simulink model "DLCI"  (R2023b)
settings: Solver=FixedStepDiscrete  StartTime=0.0  StopTime=10.0  FixedStep=0.01  RelTol=1e-3
settings Model: Creator=LENOVO-MCC  LastModifiedBy=LENOVO-MCC
settings OptimizationCC: DefaultParameterBehavior=Inlined  EnhancedBackFolding=on  PassReuseOutputArgsAs=Individual arguments  ZeroExternalMemoryAtStartup=off  ZeroInternalMemoryAtStartup=off  OptimizeBlockOrder=speed  DifferentSizesBufferReuse=on  OptimizationCustomize=off  EfficientTunableParamExpr=on
settings DebuggingCC: ParameterTunabilityLossMsg=error
settings SFSimCC: MATLABDynamicMemAlloc=off
settings RTWCC: Description=Embedded Coder  SystemTargetFile=ert.tlc  GenCodeOnly=on  TemplateMakefile=ert_default_tmf  GenerateReport=on  LaunchReport=on  GenerateCodeMetricsReport=on
settings CodeAppCC: ForceParamTrailComments=on  IgnoreCustomStorageClasses=off  OperatorAnnotations=on  SimulinkDataObjDesc=on  SFDataObjDesc=on  InsertBlockDesc=on
settings ERTTargetCC: TargetLangStandard=C99 (ISO)  GenerateSampleERTMain=on  InlinedParameterPlacement=NonHierarchical  ERTCustomFileTemplate=example_file_process.tlc

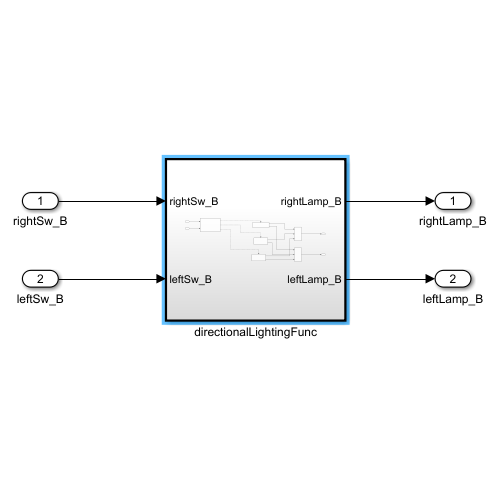
[thumbnail: Simulink's stored preview of the top-level diagram]
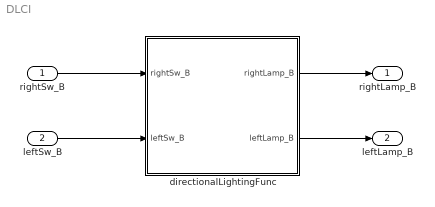
== system DLCI ==
  rightSw_B : Inport  OutDataTypeStr=boolean
  leftSw_B : Inport  Port=2  OutDataTypeStr=boolean
  directionalLightingFunc : Subsystem  TreatAsAtomicUnit=on
      settings: RTWFcnNameOpts=Use subsystem name  RTWFileNameOpts=Use subsystem name
  rightLamp_B : Outport  OutDataTypeStr=boolean
  leftLamp_B : Outport  Port=2  OutDataTypeStr=boolean
  wires:
  leftSw_B/1 -> directionalLightingFunc/2(leftSw_B)
  rightSw_B/1 -> directionalLightingFunc/1(rightSw_B)
  directionalLightingFunc/1(rightLamp_B) -> rightLamp_B/1
  directionalLightingFunc/2(leftLamp_B) -> leftLamp_B/1

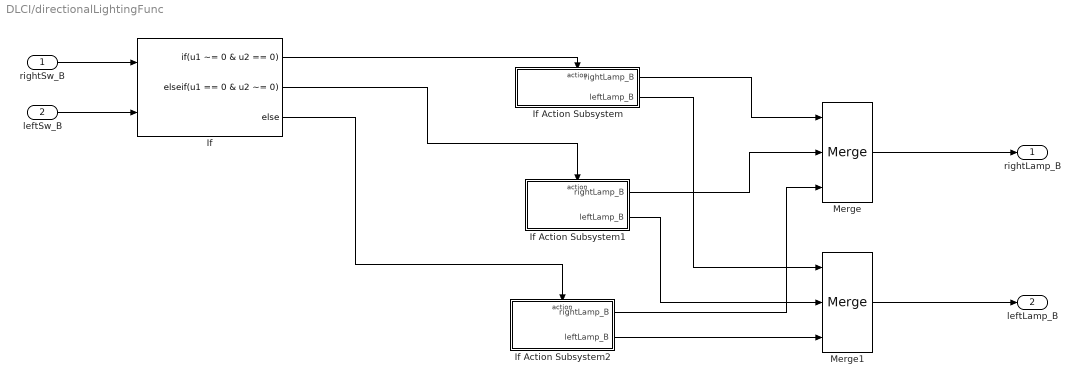
== system DLCI/directionalLightingFunc ==
  rightSw_B : Inport  OutDataTypeStr=boolean
  leftSw_B : Inport  Port=2  OutDataTypeStr=boolean
  If : If  NumInputs=2  IfExpression=u1 ~= 0 & u2 == 0  ElseIfExpressions=u1 == 0 & u2 ~= 0
  If Action Subsystem : Subsystem  TreatAsAtomicUnit=on
  If Action Subsystem1 : Subsystem  TreatAsAtomicUnit=on
  If Action Subsystem2 : Subsystem  TreatAsAtomicUnit=on
  Merge : Merge  Inputs=3
  Merge1 : Merge  Inputs=3
  rightLamp_B : Outport  OutDataTypeStr=boolean
  leftLamp_B : Outport  Port=2  OutDataTypeStr=boolean
  wires:
  rightSw_B/1 -> If/1
  leftSw_B/1 -> If/2
  If/1 -> If Action Subsystem/Action
  If/2 -> If Action Subsystem1/Action
  If/3 -> If Action Subsystem2/Action
  If Action Subsystem/1(rightLamp_B) -> Merge/1
  If Action Subsystem1/1(rightLamp_B) -> Merge/2
  If Action Subsystem2/1(rightLamp_B) -> Merge/3
  Merge/1 -> rightLamp_B/1
  Merge1/1 -> leftLamp_B/1
  If Action Subsystem/2(leftLamp_B) -> Merge1/1
  If Action Subsystem1/2(leftLamp_B) -> Merge1/2
  If Action Subsystem2/2(leftLamp_B) -> Merge1/3

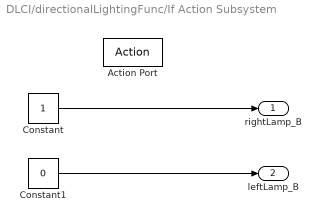
== system DLCI/directionalLightingFunc/If Action Subsystem ==
  Action Port : ActionPort  ActionPortLabel=if(u1 ~= 0 & u2 == 0)
  Constant : Constant  OutDataTypeStr=boolean
  Constant1 : Constant  Value=0  OutDataTypeStr=boolean
  rightLamp_B : Outport
  leftLamp_B : Outport  Port=2
  wires:
  Constant/1 -> rightLamp_B/1
  Constant1/1 -> leftLamp_B/1

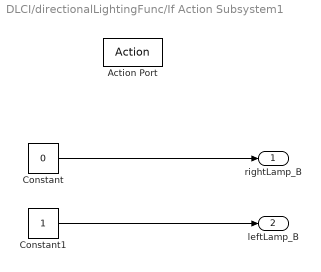
== system DLCI/directionalLightingFunc/If Action Subsystem1 ==
  Action Port : ActionPort  ActionPortLabel=elseif(u1 == 0 & u2 ~= 0)
  Constant : Constant  Value=0  OutDataTypeStr=boolean
  Constant1 : Constant  OutDataTypeStr=boolean
  rightLamp_B : Outport
  leftLamp_B : Outport  Port=2
  wires:
  Constant1/1 -> leftLamp_B/1
  Constant/1 -> rightLamp_B/1

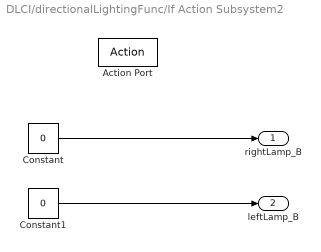
== system DLCI/directionalLightingFunc/If Action Subsystem2 ==
  Action Port : ActionPort  ActionPortLabel=else
  Constant : Constant  Value=0  OutDataTypeStr=boolean
  Constant1 : Constant  Value=0  OutDataTypeStr=boolean
  rightLamp_B : Outport
  leftLamp_B : Outport  Port=2
  wires:
  Constant1/1 -> leftLamp_B/1
  Constant/1 -> rightLamp_B/1
